simulink model "test2"  (R2015a)
settings: Solver=ode45  StartTime=0.0  StopTime=tsim  RelTol=1e-3
values from neighbouring files (symbols this model uses):
  mu = 5    [main.m]
  x1_0 = 4    [main.m]
  x2_0 = 10    [main.m]
settings Model: Creator=Martin  LastModifiedBy=Martin

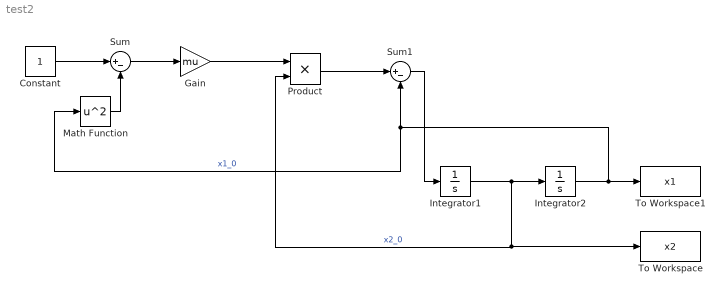
== system test2 ==
  Constant : Constant
  Gain : Gain  Gain=mu
  Integrator1 : Integrator  InitialCondition=x2_0
  Integrator2 : Integrator  InitialCondition=x1_0
  Math Function : Math  Operator=square  SaturateOnIntegerOverflow=on
  Product : Product
  Sum : Sum  Inputs=|+-
  Sum1 : Sum  Inputs=|+-
  To Workspace : ToWorkspace  VariableName=x2  SaveFormat=Timeseries  SampleTime=-1
  To Workspace1 : ToWorkspace  VariableName=x1  SaveFormat=Timeseries  SampleTime=-1
  wires:
  Constant/1 -> Sum/1
  Math Function/1 -> Sum/2
  Sum/1 -> Gain/1
  Gain/1 -> Product/1
  Product/1 -> Sum1/1
  Sum1/1 -> Integrator1/1
  Integrator1/1 -> Product/2, To Workspace/1, Integrator2/1  "x2_0"
  Integrator2/1 -> To Workspace1/1, Math Function/1, Sum1/2  "x1_0"
